simulink model "InternetServer_"  (R2019a)
settings: Solver=ode4  StartTime=0.0  StopTime=inf  FixedStep=0.01  RelTol=1e-3
libraries: SimulinkExecutionControl x1
settings Model: Creator=Tulga Ersal  LastModifiedBy=clicli
settings DataIOCC: ReturnWorkspaceOutputs=off
settings OptimizationCC: BlockReduction=off  BooleanDataType=off  LifeSpan=inf
settings DebuggingCC: SaveWithParameterizedLinksMsg=none  UnderspecifiedInitializationDetection=Classic  MergeDetectMultiDrivingBlocksExec=none  SignalResolutionControl=TryResolveAllWithWarning  SFUnexpectedBacktrackingDiag=warning  SFNoUnconditionalDefaultTransitionDiag=warning  SFExecutionAtInitializationDiag=none  ArithmeticOperatorsInVariantConditions=warning
settings HardwareCC: TargetUnknown=on
settings ModelReferenceCC: PropagateSignalLabelsOutOfModel=off
settings SFSimCC: SimUseLocalCustomCode=off
settings RTWCC: RTWUseLocalCustomCode=off
settings CodeAppCC: StateflowObjectComments=on
settings GRTTargetCC: TargetLangStandard=C89/C90 (ANSI)
settings ConfigComp: CovMetricSettings=dw  CovHtmlReporting=on  CovSaveCumulativeToWorkspaceVar=on  CovSaveSingleToWorkspaceVar=on  CovExternalEMLEnable=off

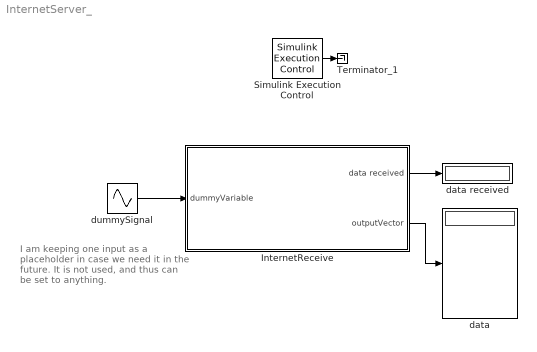
== system InternetServer_ ==
  note: I am keeping one input as a placeholder in case we need it in the future. It is not used, and thus can be set to anything.
  InternetReceive : Subsystem  mask(20-sim 4.6 S-Function block){}
      mask help:
      | This block is generated by the 20-sim Matlab Code Generator.
      |
      | * look under the mask to get information on the ports
      | * press Help for more detailed information
      | * the parameters of this block are:
      mask Help:
      | This block is generated by the 20-sim Matlab Code Generator<br>
      | The block parameters are:<br><blockquote></blockquote>
      | Generated at:<br>
      | <blockquote><b>date:  </b>June 14, 2017<br>
      | <b>time:  </b>4:16:43 PM<br></blockquote>
      | From the following 20-sim model:<br>
      | <blockquote><b>submodel:  </b>InternetServer<br>
      | <b>model:  </b>export to Simulink - UM<br>
      | <b>file:  </b>C:\Users\Tulga Ersal\Desktop\For Xueru\export to Simulink - UM.emx<br>
      | <b>experiment:  </b>C:\Users\Tulga Ersal\Desktop\For Xueru\export to Simulink - UM.emx<br></blockquote>
      | Using the following 20-sim license:<br>
      | <blockquote><b>user:  </b>The University of Michigan<br>
      | <b>from:  </b>20-sim 4.6 Student License<br>
      | <b>build: </b>4.6.1.6898<br></blockquote>
  Simulink Execution Control : SimulinkExecutionControl/Simulink Execution Control  proc_pri=REALTIME_PRIORITY_CLASS  thread_pri=THREAD_PRIORITY_TIME_CRITICAL  rt_sim=on  factor=1  ovrrun=Continue execution  Ts=0.01
  Terminator_1 : Terminator
  data : Display
  data received : Display
  dummySignal : Sin  SampleTime=0
  wires:
  Simulink Execution Control/1 -> Terminator_1/1
  dummySignal/1 -> InternetReceive/1(dummyVariable)
  InternetReceive/1(data received) -> data received/1
  InternetReceive/2(outputVector) -> data/1

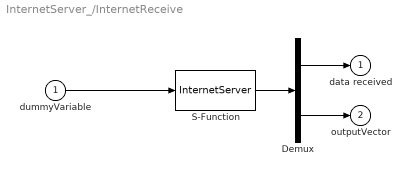
== system InternetServer_/InternetReceive ==
  dummyVariable : Inport
  Demux : Demux  Outputs=[1 -1]
  S-Function : S-Function  FunctionName=InternetServer  SFunctionDeploymentMode=off  EnableBusSupport=off
  data received : Outport
  outputVector : Outport  Port=2
  wires:
  dummyVariable/1 -> S-Function/1
  S-Function/1 -> Demux/1
  Demux/1 -> data received/1
  Demux/2 -> outputVector/1
